simulink model "Brakes"  (R2014a)
settings: Solver=ode45  StartTime=0.0  StopTime=10.0  RelTol=1e-3
model workspace: external: MAT-File Vehicle\Brakes\Data\Brakes.mat (data not in the file)
undefined symbols (not defined in the file): kb, ub
settings Model: Creator=Nathan  LastModifiedBy=Nathan
settings OptimizationCC: InlineParams=on
settings DebuggingCC: UnderspecifiedInitializationDetection=Classic  StateNameClashWarn=warning
settings ModelReferenceCC: ModelReferenceMinAlgLoopOccurrences=on

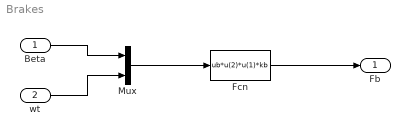
== system Brakes ==
  Beta : Inport
  wt : Inport  Port=2
  Fcn : Fcn  Expr=ub*u(2)*u(1)*kb
  Mux : Mux  Inputs=2
  Fb : Outport
  wires:
  Beta/1 -> Mux/1
  wt/1 -> Mux/2
  Fcn/1 -> Fb/1
  Mux/1 -> Fcn/1
